simulink model "rootlocus2"  (R2016a)
settings: Solver=VariableStepAuto  StartTime=0.0  StopTime=10  RelTol=1e-3
values from neighbouring files (symbols this model uses):
  den_K1 = [1 2 1]    [rootlocus.m]
  den_K2 = [1 10 25]    [rootlocus.m]
  K1 = 1    [rootlocus.m]
  K2 = 9    [rootlocus.m]
  num_K1 = [2]    [rootlocus.m]
  num_K2 = [2]    [rootlocus.m]
libraries: simulink x3
settings Model: Creator=73565  LastModifiedBy=Administrator

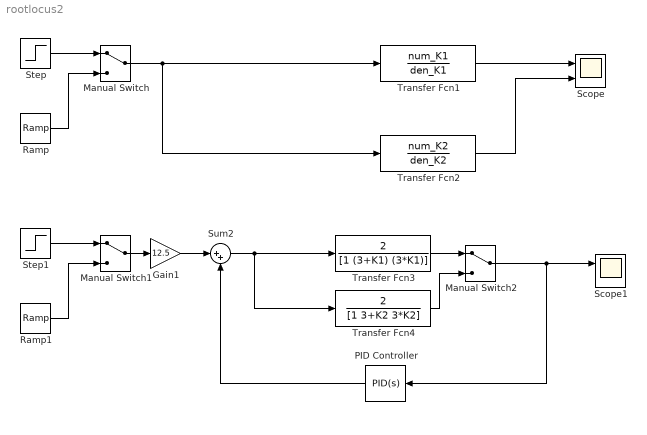
== system rootlocus2 ==
  Gain1 : Gain  Gain=12.5
  Manual Switch : ManualSwitch
  Manual Switch1 : ManualSwitch
  Manual Switch2 : ManualSwitch
  PID Controller : simulink/Continuous/PID Controller  Controller=PID  TimeDomain=Continuous-time  SampleTime=-1  IntegratorMethod=Forward Euler  FilterMethod=Forward Euler  Form=Parallel  UseFilter=on  ControllerParametersSource=internal  P=1  I=0  D=1  N=100  InitialConditionSource=internal  InitialConditionForIntegrator=0  InitialConditionForFilter=0  ExternalReset=none  LimitOutput=off  UpperSaturationLimit=inf  LowerSaturationLimit=-inf  LinearizeAsGain=on  AntiWindupMode=none  Kb=1  TrackingMode=off  Kt=1  PParamMin=[]  PParamMax=[]  IParamMin=[]  IParamMax=[]  DParamMin=[]  DParamMax=[]  NParamMin=[]  NParamMax=[]  KbParamMin=[]  KbParamMax=[]  KtParamMin=[]  KtParamMax=[]  POutMin=[]  POutMax=[]  IOutMin=[]  IOutMax=[]  DOutMin=[]  DOutMax=[]  NOutMin=[]  NOutMax=[]  KbOutMin=[]  KbOutMax=[]  KtOutMin=[]  KtOutMax=[]  IntegratorOutMin=[]  IntegratorOutMax=[]  FilterOutMin=[]  FilterOutMax=[]  SumOutMin=[]  SumOutMax=[]  SumI1OutMin=[]  SumI1OutMax=[]  SumI2OutMin=[]  SumI2OutMax=[]  SumI3OutMin=[]  SumI3OutMax=[]  SumDOutMin=[]  SumDOutMax=[]  SaturationOutMin=[]  SaturationOutMax=[]  IntegratorContinuousStateAttributes=''  IntegratorStateMustResolveToSignalObject=off  IntegratorRTWStateStorageClass=Auto  FilterContinuousStateAttributes=''  FilterStateMustResolveToSignalObject=off  FilterRTWStateStorageClass=Auto  DifferentiatorICPrevScaledInput=0  DifferentiatorOutMin=[]  DifferentiatorOutMax=[]
  Ramp : simulink/Sources/Ramp  slope=1  start=0  X0=0
  Ramp1 : simulink/Sources/Ramp  slope=1  start=0  X0=0
  Scope : Scope  NumInputPorts=2
  Scope1 : Scope  NumInputPorts=2
  Step : Step  SampleTime=0
  Step1 : Step  SampleTime=0
  Sum2 : Sum  Inputs=|++
  Transfer Fcn1 : TransferFcn  Numerator=num_K1  Denominator=den_K1
  Transfer Fcn2 : TransferFcn  Numerator=num_K2  Denominator=den_K2
  Transfer Fcn3 : TransferFcn  Numerator=[2]  Denominator=[1 (3+K1) (3*K1)]
  Transfer Fcn4 : TransferFcn  Numerator=[2]  Denominator=[1 3+K2 3*K2]
  wires:
  Manual Switch/1 -> Transfer Fcn1/1, Transfer Fcn2/1
  Transfer Fcn1/1 -> Scope/1
  Step/1 -> Manual Switch/1
  Ramp/1 -> Manual Switch/2
  Transfer Fcn2/1 -> Scope/2
  Step1/1 -> Manual Switch1/1
  Ramp1/1 -> Manual Switch1/2
  PID Controller/1 -> Sum2/2
  Transfer Fcn3/1 -> Manual Switch2/1
  Manual Switch2/1 -> PID Controller/1, Scope1/1
  Transfer Fcn4/1 -> Manual Switch2/2
  Sum2/1 -> Transfer Fcn3/1, Transfer Fcn4/1
  Manual Switch1/1 -> Gain1/1
  Gain1/1 -> Sum2/1
